simulink model "c00014M_harness"  (R2018a)
settings: Solver=ode3  StartTime=0.0  StopTime=10.0  RelTol=1e-3  EnableMultiTasking=on
undefined symbols (not defined in the file): b, DiscIntNeverNeededParam, J, K, L, PosMinimaW4, R, sigbuilder_block
(part 8 of 46)

== system c00014M_harness/M090 ==
  DW1 : Inport  OutMin=0  OutMax=4  OutDataTypeStr=int8
  DW2 : Inport  Port=2  OutMin=0  OutMax=4  OutDataTypeStr=int8
  DW4 : Inport  Port=3  OutMin=0  OutMax=4  OutDataTypeStr=int8
  P1W2 : Inport  Port=4  OutMin=0  OutMax=4  OutDataTypeStr=int8
  P3W4 : Inport  Port=5  OutMin=0  OutMax=4  OutDataTypeStr=int8
  P1W4 : Inport  Port=6  OutMin=0  OutMax=4  OutDataTypeStr=int8
  O1 : Inport  Port=7  OutDataTypeStr=boolean
  O2 : Inport  Port=8  OutDataTypeStr=boolean
  O4 : Inport  Port=9  OutDataTypeStr=boolean
  LD : Inport  Port=10  OutDataTypeStr=boolean
  CW1C : Inport  Port=11  OutMin=0  OutMax=4  OutDataTypeStr=int8
  CW2C : Inport  Port=12  OutMin=0  OutMax=4  OutDataTypeStr=int8
  CW4C : Inport  Port=13  OutMin=0  OutMax=4  OutDataTypeStr=int8
  Cyber : Subsystem
  M : Memory
  M1 : Memory
  M3 : Memory
  Physical : Subsystem
  S1 : Subsystem
  S2 : Subsystem
  S4 : Subsystem
  W1Pos : Outport
  W2Pos : Outport  Port=2
  W4Pos : Outport  Port=3
  wires:
  Cyber/3(W4) -> Physical/3(InW4)
  DW4/1 -> Cyber/6(DW4)
  Physical/3(W4) -> S4/1(PhyMeasure), W4Pos/1
  DW2/1 -> Cyber/5(DW2)
  P3W4/1 -> Cyber/8(P3W4)
  S2/1(SensorOut) -> M1/1
  Physical/2(W2) -> S2/1(PhyMeasure), W2Pos/1
  DW1/1 -> Cyber/4(DW1)
  M/1 -> Cyber/1(PosW1)
  M1/1 -> Cyber/2(PosW2)
  S4/1(SensorOut) -> M3/1
  CW1C/1 -> Cyber/14(CW1C)
  P1W4/1 -> Cyber/9(P1W4)
  P1W2/1 -> Cyber/7(P1W2)
  Cyber/2(W2) -> Physical/2(InW2)
  Cyber/1(W1) -> Physical/1(InW1)
  O1/1 -> Cyber/10(OW1)
  LD/1 -> Cyber/13(LD)
  O2/1 -> Cyber/11(OW2)
  O4/1 -> Cyber/12(OW4)
  Physical/1(W1) -> S1/1(PhyMeasure), W1Pos/1
  CW4C/1 -> Cyber/16(CW4C)
  CW2C/1 -> Cyber/15(CW2C)
  S1/1(SensorOut) -> M/1
  M3/1 -> Cyber/3(PosW4)

== system c00014M_harness/M091 ==
  DW1 : Inport  OutMin=0  OutMax=4  OutDataTypeStr=int8
  DW2 : Inport  Port=2  OutMin=0  OutMax=4  OutDataTypeStr=int8
  DW4 : Inport  Port=3  OutMin=0  OutMax=4  OutDataTypeStr=int8
  P1W2 : Inport  Port=4  OutMin=0  OutMax=4  OutDataTypeStr=int8
  P3W4 : Inport  Port=5  OutMin=0  OutMax=4  OutDataTypeStr=int8
  P1W4 : Inport  Port=6  OutMin=0  OutMax=4  OutDataTypeStr=int8
  O1 : Inport  Port=7  OutDataTypeStr=boolean
  O2 : Inport  Port=8  OutDataTypeStr=boolean
  O4 : Inport  Port=9  OutDataTypeStr=boolean
  LD : Inport  Port=10  OutDataTypeStr=boolean
  CW1C : Inport  Port=11  OutMin=0  OutMax=4  OutDataTypeStr=int8
  CW2C : Inport  Port=12  OutMin=0  OutMax=4  OutDataTypeStr=int8
  CW4C : Inport  Port=13  OutMin=0  OutMax=4  OutDataTypeStr=int8
  Cyber : Subsystem
  M : Memory
  M1 : Memory
  M3 : Memory
  Physical : Subsystem
  S1 : Subsystem
  S2 : Subsystem
  S4 : Subsystem
  W1Pos : Outport
  W2Pos : Outport  Port=2
  W4Pos : Outport  Port=3
  wires:
  Cyber/3(W4) -> Physical/3(InW4)
  DW4/1 -> Cyber/6(DW4)
  Physical/3(W4) -> S4/1(PhyMeasure), W4Pos/1
  DW2/1 -> Cyber/5(DW2)
  P3W4/1 -> Cyber/8(P3W4)
  S2/1(SensorOut) -> M1/1
  Physical/2(W2) -> S2/1(PhyMeasure), W2Pos/1
  DW1/1 -> Cyber/4(DW1)
  M/1 -> Cyber/1(PosW1)
  M1/1 -> Cyber/2(PosW2)
  S4/1(SensorOut) -> M3/1
  CW1C/1 -> Cyber/14(CW1C)
  P1W4/1 -> Cyber/9(P1W4)
  P1W2/1 -> Cyber/7(P1W2)
  Cyber/2(W2) -> Physical/2(InW2)
  Cyber/1(W1) -> Physical/1(InW1)
  O1/1 -> Cyber/10(OW1)
  LD/1 -> Cyber/13(LD)
  O2/1 -> Cyber/11(OW2)
  O4/1 -> Cyber/12(OW4)
  Physical/1(W1) -> S1/1(PhyMeasure), W1Pos/1
  CW4C/1 -> Cyber/16(CW4C)
  CW2C/1 -> Cyber/15(CW2C)
  S1/1(SensorOut) -> M/1
  M3/1 -> Cyber/3(PosW4)

== system c00014M_harness/M092 ==
  DW1 : Inport  OutMin=0  OutMax=4  OutDataTypeStr=int8
  DW2 : Inport  Port=2  OutMin=0  OutMax=4  OutDataTypeStr=int8
  DW4 : Inport  Port=3  OutMin=0  OutMax=4  OutDataTypeStr=int8
  P1W2 : Inport  Port=4  OutMin=0  OutMax=4  OutDataTypeStr=int8
  P3W4 : Inport  Port=5  OutMin=0  OutMax=4  OutDataTypeStr=int8
  P1W4 : Inport  Port=6  OutMin=0  OutMax=4  OutDataTypeStr=int8
  O1 : Inport  Port=7  OutDataTypeStr=boolean
  O2 : Inport  Port=8  OutDataTypeStr=boolean
  O4 : Inport  Port=9  OutDataTypeStr=boolean
  LD : Inport  Port=10  OutDataTypeStr=boolean
  CW1C : Inport  Port=11  OutMin=0  OutMax=4  OutDataTypeStr=int8
  CW2C : Inport  Port=12  OutMin=0  OutMax=4  OutDataTypeStr=int8
  CW4C : Inport  Port=13  OutMin=0  OutMax=4  OutDataTypeStr=int8
  Cyber : Subsystem
  M : Memory
  M1 : Memory
  M3 : Memory
  Physical : Subsystem
  S1 : Subsystem
  S2 : Subsystem
  S4 : Subsystem
  W1Pos : Outport
  W2Pos : Outport  Port=2
  W4Pos : Outport  Port=3
  wires:
  Cyber/3(W4) -> Physical/3(InW4)
  DW4/1 -> Cyber/6(DW4)
  Physical/3(W4) -> S4/1(PhyMeasure), W4Pos/1
  DW2/1 -> Cyber/5(DW2)
  P3W4/1 -> Cyber/8(P3W4)
  S2/1(SensorOut) -> M1/1
  Physical/2(W2) -> S2/1(PhyMeasure), W2Pos/1
  DW1/1 -> Cyber/4(DW1)
  M/1 -> Cyber/1(PosW1)
  M1/1 -> Cyber/2(PosW2)
  S4/1(SensorOut) -> M3/1
  CW1C/1 -> Cyber/14(CW1C)
  P1W4/1 -> Cyber/9(P1W4)
  P1W2/1 -> Cyber/7(P1W2)
  Cyber/2(W2) -> Physical/2(InW2)
  Cyber/1(W1) -> Physical/1(InW1)
  O1/1 -> Cyber/10(OW1)
  LD/1 -> Cyber/13(LD)
  O2/1 -> Cyber/11(OW2)
  O4/1 -> Cyber/12(OW4)
  Physical/1(W1) -> S1/1(PhyMeasure), W1Pos/1
  CW4C/1 -> Cyber/16(CW4C)
  CW2C/1 -> Cyber/15(CW2C)
  S1/1(SensorOut) -> M/1
  M3/1 -> Cyber/3(PosW4)

== system c00014M_harness/M094 ==
  DW1 : Inport  OutMin=0  OutMax=4  OutDataTypeStr=int8
  DW2 : Inport  Port=2  OutMin=0  OutMax=4  OutDataTypeStr=int8
  DW4 : Inport  Port=3  OutMin=0  OutMax=4  OutDataTypeStr=int8
  P1W2 : Inport  Port=4  OutMin=0  OutMax=4  OutDataTypeStr=int8
  P3W4 : Inport  Port=5  OutMin=0  OutMax=4  OutDataTypeStr=int8
  P1W4 : Inport  Port=6  OutMin=0  OutMax=4  OutDataTypeStr=int8
  O1 : Inport  Port=7  OutDataTypeStr=boolean
  O2 : Inport  Port=8  OutDataTypeStr=boolean
  O4 : Inport  Port=9  OutDataTypeStr=boolean
  LD : Inport  Port=10  OutDataTypeStr=boolean
  CW1C : Inport  Port=11  OutMin=0  OutMax=4  OutDataTypeStr=int8
  CW2C : Inport  Port=12  OutMin=0  OutMax=4  OutDataTypeStr=int8
  CW4C : Inport  Port=13  OutMin=0  OutMax=4  OutDataTypeStr=int8
  Cyber : Subsystem
  M : Memory
  M1 : Memory
  M3 : Memory
  Physical : Subsystem
  S1 : Subsystem
  S2 : Subsystem
  S4 : Subsystem
  W1Pos : Outport
  W2Pos : Outport  Port=2
  W4Pos : Outport  Port=3
  wires:
  Cyber/3(W4) -> Physical/3(InW4)
  DW4/1 -> Cyber/6(DW4)
  Physical/3(W4) -> S4/1(PhyMeasure), W4Pos/1
  DW2/1 -> Cyber/5(DW2)
  P3W4/1 -> Cyber/8(P3W4)
  S2/1(SensorOut) -> M1/1
  Physical/2(W2) -> S2/1(PhyMeasure), W2Pos/1
  DW1/1 -> Cyber/4(DW1)
  M/1 -> Cyber/1(PosW1)
  M1/1 -> Cyber/2(PosW2)
  S4/1(SensorOut) -> M3/1
  CW1C/1 -> Cyber/14(CW1C)
  P1W4/1 -> Cyber/9(P1W4)
  P1W2/1 -> Cyber/7(P1W2)
  Cyber/2(W2) -> Physical/2(InW2)
  Cyber/1(W1) -> Physical/1(InW1)
  O1/1 -> Cyber/10(OW1)
  LD/1 -> Cyber/13(LD)
  O2/1 -> Cyber/11(OW2)
  O4/1 -> Cyber/12(OW4)
  Physical/1(W1) -> S1/1(PhyMeasure), W1Pos/1
  CW4C/1 -> Cyber/16(CW4C)
  CW2C/1 -> Cyber/15(CW2C)
  S1/1(SensorOut) -> M/1
  M3/1 -> Cyber/3(PosW4)

== system c00014M_harness/M095 ==
  DW1 : Inport  OutMin=0  OutMax=4  OutDataTypeStr=int8
  DW2 : Inport  Port=2  OutMin=0  OutMax=4  OutDataTypeStr=int8
  DW4 : Inport  Port=3  OutMin=0  OutMax=4  OutDataTypeStr=int8
  P1W2 : Inport  Port=4  OutMin=0  OutMax=4  OutDataTypeStr=int8
  P3W4 : Inport  Port=5  OutMin=0  OutMax=4  OutDataTypeStr=int8
  P1W4 : Inport  Port=6  OutMin=0  OutMax=4  OutDataTypeStr=int8
  O1 : Inport  Port=7  OutDataTypeStr=boolean
  O2 : Inport  Port=8  OutDataTypeStr=boolean
  O4 : Inport  Port=9  OutDataTypeStr=boolean
  LD : Inport  Port=10  OutDataTypeStr=boolean
  CW1C : Inport  Port=11  OutMin=0  OutMax=4  OutDataTypeStr=int8
  CW2C : Inport  Port=12  OutMin=0  OutMax=4  OutDataTypeStr=int8
  CW4C : Inport  Port=13  OutMin=0  OutMax=4  OutDataTypeStr=int8
  Cyber : Subsystem
  M : Memory
  M1 : Memory
  M3 : Memory
  Physical : Subsystem
  S1 : Subsystem
  S2 : Subsystem
  S4 : Subsystem
  W1Pos : Outport
  W2Pos : Outport  Port=2
  W4Pos : Outport  Port=3
  wires:
  Cyber/3(W4) -> Physical/3(InW4)
  DW4/1 -> Cyber/6(DW4)
  Physical/3(W4) -> S4/1(PhyMeasure), W4Pos/1
  DW2/1 -> Cyber/5(DW2)
  P3W4/1 -> Cyber/8(P3W4)
  S2/1(SensorOut) -> M1/1
  Physical/2(W2) -> S2/1(PhyMeasure), W2Pos/1
  DW1/1 -> Cyber/4(DW1)
  M/1 -> Cyber/1(PosW1)
  M1/1 -> Cyber/2(PosW2)
  S4/1(SensorOut) -> M3/1
  CW1C/1 -> Cyber/14(CW1C)
  P1W4/1 -> Cyber/9(P1W4)
  P1W2/1 -> Cyber/7(P1W2)
  Cyber/2(W2) -> Physical/2(InW2)
  Cyber/1(W1) -> Physical/1(InW1)
  O1/1 -> Cyber/10(OW1)
  LD/1 -> Cyber/13(LD)
  O2/1 -> Cyber/11(OW2)
  O4/1 -> Cyber/12(OW4)
  Physical/1(W1) -> S1/1(PhyMeasure), W1Pos/1
  CW4C/1 -> Cyber/16(CW4C)
  CW2C/1 -> Cyber/15(CW2C)
  S1/1(SensorOut) -> M/1
  M3/1 -> Cyber/3(PosW4)

== system c00014M_harness/M096 ==
  DW1 : Inport  OutMin=0  OutMax=4  OutDataTypeStr=int8
  DW2 : Inport  Port=2  OutMin=0  OutMax=4  OutDataTypeStr=int8
  DW4 : Inport  Port=3  OutMin=0  OutMax=4  OutDataTypeStr=int8
  P1W2 : Inport  Port=4  OutMin=0  OutMax=4  OutDataTypeStr=int8
  P3W4 : Inport  Port=5  OutMin=0  OutMax=4  OutDataTypeStr=int8
  P1W4 : Inport  Port=6  OutMin=0  OutMax=4  OutDataTypeStr=int8
  O1 : Inport  Port=7  OutDataTypeStr=boolean
  O2 : Inport  Port=8  OutDataTypeStr=boolean
  O4 : Inport  Port=9  OutDataTypeStr=boolean
  LD : Inport  Port=10  OutDataTypeStr=boolean
  CW1C : Inport  Port=11  OutMin=0  OutMax=4  OutDataTypeStr=int8
  CW2C : Inport  Port=12  OutMin=0  OutMax=4  OutDataTypeStr=int8
  CW4C : Inport  Port=13  OutMin=0  OutMax=4  OutDataTypeStr=int8
  Cyber : Subsystem
  M : Memory
  M1 : Memory
  M3 : Memory
  Physical : Subsystem
  S1 : Subsystem
  S2 : Subsystem
  S4 : Subsystem
  W1Pos : Outport
  W2Pos : Outport  Port=2
  W4Pos : Outport  Port=3
  wires:
  Cyber/3(W4) -> Physical/3(InW4)
  DW4/1 -> Cyber/6(DW4)
  Physical/3(W4) -> S4/1(PhyMeasure), W4Pos/1
  DW2/1 -> Cyber/5(DW2)
  P3W4/1 -> Cyber/8(P3W4)
  S2/1(SensorOut) -> M1/1
  Physical/2(W2) -> S2/1(PhyMeasure), W2Pos/1
  DW1/1 -> Cyber/4(DW1)
  M/1 -> Cyber/1(PosW1)
  M1/1 -> Cyber/2(PosW2)
  S4/1(SensorOut) -> M3/1
  CW1C/1 -> Cyber/14(CW1C)
  P1W4/1 -> Cyber/9(P1W4)
  P1W2/1 -> Cyber/7(P1W2)
  Cyber/2(W2) -> Physical/2(InW2)
  Cyber/1(W1) -> Physical/1(InW1)
  O1/1 -> Cyber/10(OW1)
  LD/1 -> Cyber/13(LD)
  O2/1 -> Cyber/11(OW2)
  O4/1 -> Cyber/12(OW4)
  Physical/1(W1) -> S1/1(PhyMeasure), W1Pos/1
  CW4C/1 -> Cyber/16(CW4C)
  CW2C/1 -> Cyber/15(CW2C)
  S1/1(SensorOut) -> M/1
  M3/1 -> Cyber/3(PosW4)

== system c00014M_harness/M098 ==
  DW1 : Inport  OutMin=0  OutMax=4  OutDataTypeStr=int8
  DW2 : Inport  Port=2  OutMin=0  OutMax=4  OutDataTypeStr=int8
  DW4 : Inport  Port=3  OutMin=0  OutMax=4  OutDataTypeStr=int8
  P1W2 : Inport  Port=4  OutMin=0  OutMax=4  OutDataTypeStr=int8
  P3W4 : Inport  Port=5  OutMin=0  OutMax=4  OutDataTypeStr=int8
  P1W4 : Inport  Port=6  OutMin=0  OutMax=4  OutDataTypeStr=int8
  O1 : Inport  Port=7  OutDataTypeStr=boolean
  O2 : Inport  Port=8  OutDataTypeStr=boolean
  O4 : Inport  Port=9  OutDataTypeStr=boolean
  LD : Inport  Port=10  OutDataTypeStr=boolean
  CW1C : Inport  Port=11  OutMin=0  OutMax=4  OutDataTypeStr=int8
  CW2C : Inport  Port=12  OutMin=0  OutMax=4  OutDataTypeStr=int8
  CW4C : Inport  Port=13  OutMin=0  OutMax=4  OutDataTypeStr=int8
  Cyber : Subsystem
  M : Memory
  M1 : Memory
  M3 : Memory
  Physical : Subsystem
  S1 : Subsystem
  S2 : Subsystem
  S4 : Subsystem
  W1Pos : Outport
  W2Pos : Outport  Port=2
  W4Pos : Outport  Port=3
  wires:
  Cyber/3(W4) -> Physical/3(InW4)
  DW4/1 -> Cyber/6(DW4)
  Physical/3(W4) -> S4/1(PhyMeasure), W4Pos/1
  DW2/1 -> Cyber/5(DW2)
  P3W4/1 -> Cyber/8(P3W4)
  S2/1(SensorOut) -> M1/1
  Physical/2(W2) -> S2/1(PhyMeasure), W2Pos/1
  DW1/1 -> Cyber/4(DW1)
  M/1 -> Cyber/1(PosW1)
  M1/1 -> Cyber/2(PosW2)
  S4/1(SensorOut) -> M3/1
  CW1C/1 -> Cyber/14(CW1C)
  P1W4/1 -> Cyber/9(P1W4)
  P1W2/1 -> Cyber/7(P1W2)
  Cyber/2(W2) -> Physical/2(InW2)
  Cyber/1(W1) -> Physical/1(InW1)
  O1/1 -> Cyber/10(OW1)
  LD/1 -> Cyber/13(LD)
  O2/1 -> Cyber/11(OW2)
  O4/1 -> Cyber/12(OW4)
  Physical/1(W1) -> S1/1(PhyMeasure), W1Pos/1
  CW4C/1 -> Cyber/16(CW4C)
  CW2C/1 -> Cyber/15(CW2C)
  S1/1(SensorOut) -> M/1
  M3/1 -> Cyber/3(PosW4)

== system c00014M_harness/M099 ==
  DW1 : Inport  OutMin=0  OutMax=4  OutDataTypeStr=int8
  DW2 : Inport  Port=2  OutMin=0  OutMax=4  OutDataTypeStr=int8
  DW4 : Inport  Port=3  OutMin=0  OutMax=4  OutDataTypeStr=int8
  P1W2 : Inport  Port=4  OutMin=0  OutMax=4  OutDataTypeStr=int8
  P3W4 : Inport  Port=5  OutMin=0  OutMax=4  OutDataTypeStr=int8
  P1W4 : Inport  Port=6  OutMin=0  OutMax=4  OutDataTypeStr=int8
  O1 : Inport  Port=7  OutDataTypeStr=boolean
  O2 : Inport  Port=8  OutDataTypeStr=boolean
  O4 : Inport  Port=9  OutDataTypeStr=boolean
  LD : Inport  Port=10  OutDataTypeStr=boolean
  CW1C : Inport  Port=11  OutMin=0  OutMax=4  OutDataTypeStr=int8
  CW2C : Inport  Port=12  OutMin=0  OutMax=4  OutDataTypeStr=int8
  CW4C : Inport  Port=13  OutMin=0  OutMax=4  OutDataTypeStr=int8
  Cyber : Subsystem
  M : Memory
  M1 : Memory
  M3 : Memory
  Physical : Subsystem
  S1 : Subsystem
  S2 : Subsystem
  S4 : Subsystem
  W1Pos : Outport
  W2Pos : Outport  Port=2
  W4Pos : Outport  Port=3
  wires:
  Cyber/3(W4) -> Physical/3(InW4)
  DW4/1 -> Cyber/6(DW4)
  Physical/3(W4) -> S4/1(PhyMeasure), W4Pos/1
  DW2/1 -> Cyber/5(DW2)
  P3W4/1 -> Cyber/8(P3W4)
  S2/1(SensorOut) -> M1/1
  Physical/2(W2) -> S2/1(PhyMeasure), W2Pos/1
  DW1/1 -> Cyber/4(DW1)
  M/1 -> Cyber/1(PosW1)
  M1/1 -> Cyber/2(PosW2)
  S4/1(SensorOut) -> M3/1
  CW1C/1 -> Cyber/14(CW1C)
  P1W4/1 -> Cyber/9(P1W4)
  P1W2/1 -> Cyber/7(P1W2)
  Cyber/2(W2) -> Physical/2(InW2)
  Cyber/1(W1) -> Physical/1(InW1)
  O1/1 -> Cyber/10(OW1)
  LD/1 -> Cyber/13(LD)
  O2/1 -> Cyber/11(OW2)
  O4/1 -> Cyber/12(OW4)
  Physical/1(W1) -> S1/1(PhyMeasure), W1Pos/1
  CW4C/1 -> Cyber/16(CW4C)
  CW2C/1 -> Cyber/15(CW2C)
  S1/1(SensorOut) -> M/1
  M3/1 -> Cyber/3(PosW4)

== system c00014M_harness/M100 ==
  DW1 : Inport  OutMin=0  OutMax=4  OutDataTypeStr=int8
  DW2 : Inport  Port=2  OutMin=0  OutMax=4  OutDataTypeStr=int8
  DW4 : Inport  Port=3  OutMin=0  OutMax=4  OutDataTypeStr=int8
  P1W2 : Inport  Port=4  OutMin=0  OutMax=4  OutDataTypeStr=int8
  P3W4 : Inport  Port=5  OutMin=0  OutMax=4  OutDataTypeStr=int8
  P1W4 : Inport  Port=6  OutMin=0  OutMax=4  OutDataTypeStr=int8
  O1 : Inport  Port=7  OutDataTypeStr=boolean
  O2 : Inport  Port=8  OutDataTypeStr=boolean
  O4 : Inport  Port=9  OutDataTypeStr=boolean
  LD : Inport  Port=10  OutDataTypeStr=boolean
  CW1C : Inport  Port=11  OutMin=0  OutMax=4  OutDataTypeStr=int8
  CW2C : Inport  Port=12  OutMin=0  OutMax=4  OutDataTypeStr=int8
  CW4C : Inport  Port=13  OutMin=0  OutMax=4  OutDataTypeStr=int8
  Cyber : Subsystem
  M : Memory
  M1 : Memory
  M3 : Memory
  Physical : Subsystem
  S1 : Subsystem
  S2 : Subsystem
  S4 : Subsystem
  W1Pos : Outport
  W2Pos : Outport  Port=2
  W4Pos : Outport  Port=3
  wires:
  Cyber/3(W4) -> Physical/3(InW4)
  DW4/1 -> Cyber/6(DW4)
  Physical/3(W4) -> S4/1(PhyMeasure), W4Pos/1
  DW2/1 -> Cyber/5(DW2)
  P3W4/1 -> Cyber/8(P3W4)
  S2/1(SensorOut) -> M1/1
  Physical/2(W2) -> S2/1(PhyMeasure), W2Pos/1
  DW1/1 -> Cyber/4(DW1)
  M/1 -> Cyber/1(PosW1)
  M1/1 -> Cyber/2(PosW2)
  S4/1(SensorOut) -> M3/1
  CW1C/1 -> Cyber/14(CW1C)
  P1W4/1 -> Cyber/9(P1W4)
  P1W2/1 -> Cyber/7(P1W2)
  Cyber/2(W2) -> Physical/2(InW2)
  Cyber/1(W1) -> Physical/1(InW1)
  O1/1 -> Cyber/10(OW1)
  LD/1 -> Cyber/13(LD)
  O2/1 -> Cyber/11(OW2)
  O4/1 -> Cyber/12(OW4)
  Physical/1(W1) -> S1/1(PhyMeasure), W1Pos/1
  CW4C/1 -> Cyber/16(CW4C)
  CW2C/1 -> Cyber/15(CW2C)
  S1/1(SensorOut) -> M/1
  M3/1 -> Cyber/3(PosW4)

== system c00014M_harness/M102 ==
  DW1 : Inport  OutMin=0  OutMax=4  OutDataTypeStr=int8
  DW2 : Inport  Port=2  OutMin=0  OutMax=4  OutDataTypeStr=int8
  DW4 : Inport  Port=3  OutMin=0  OutMax=4  OutDataTypeStr=int8
  P1W2 : Inport  Port=4  OutMin=0  OutMax=4  OutDataTypeStr=int8
  P3W4 : Inport  Port=5  OutMin=0  OutMax=4  OutDataTypeStr=int8
  P1W4 : Inport  Port=6  OutMin=0  OutMax=4  OutDataTypeStr=int8
  O1 : Inport  Port=7  OutDataTypeStr=boolean
  O2 : Inport  Port=8  OutDataTypeStr=boolean
  O4 : Inport  Port=9  OutDataTypeStr=boolean
  LD : Inport  Port=10  OutDataTypeStr=boolean
  CW1C : Inport  Port=11  OutMin=0  OutMax=4  OutDataTypeStr=int8
  CW2C : Inport  Port=12  OutMin=0  OutMax=4  OutDataTypeStr=int8
  CW4C : Inport  Port=13  OutMin=0  OutMax=4  OutDataTypeStr=int8
  Cyber : Subsystem
  M : Memory
  M1 : Memory
  M3 : Memory
  Physical : Subsystem
  S1 : Subsystem
  S2 : Subsystem
  S4 : Subsystem
  W1Pos : Outport
  W2Pos : Outport  Port=2
  W4Pos : Outport  Port=3
  wires:
  Cyber/3(W4) -> Physical/3(InW4)
  DW4/1 -> Cyber/6(DW4)
  Physical/3(W4) -> S4/1(PhyMeasure), W4Pos/1
  DW2/1 -> Cyber/5(DW2)
  P3W4/1 -> Cyber/8(P3W4)
  S2/1(SensorOut) -> M1/1
  Physical/2(W2) -> S2/1(PhyMeasure), W2Pos/1
  DW1/1 -> Cyber/4(DW1)
  M/1 -> Cyber/1(PosW1)
  M1/1 -> Cyber/2(PosW2)
  S4/1(SensorOut) -> M3/1
  CW1C/1 -> Cyber/14(CW1C)
  P1W4/1 -> Cyber/9(P1W4)
  P1W2/1 -> Cyber/7(P1W2)
  Cyber/2(W2) -> Physical/2(InW2)
  Cyber/1(W1) -> Physical/1(InW1)
  O1/1 -> Cyber/10(OW1)
  LD/1 -> Cyber/13(LD)
  O2/1 -> Cyber/11(OW2)
  O4/1 -> Cyber/12(OW4)
  Physical/1(W1) -> S1/1(PhyMeasure), W1Pos/1
  CW4C/1 -> Cyber/16(CW4C)
  CW2C/1 -> Cyber/15(CW2C)
  S1/1(SensorOut) -> M/1
  M3/1 -> Cyber/3(PosW4)

== system c00014M_harness/M103 ==
  DW1 : Inport  OutMin=0  OutMax=4  OutDataTypeStr=int8
  DW2 : Inport  Port=2  OutMin=0  OutMax=4  OutDataTypeStr=int8
  DW4 : Inport  Port=3  OutMin=0  OutMax=4  OutDataTypeStr=int8
  P1W2 : Inport  Port=4  OutMin=0  OutMax=4  OutDataTypeStr=int8
  P3W4 : Inport  Port=5  OutMin=0  OutMax=4  OutDataTypeStr=int8
  P1W4 : Inport  Port=6  OutMin=0  OutMax=4  OutDataTypeStr=int8
  O1 : Inport  Port=7  OutDataTypeStr=boolean
  O2 : Inport  Port=8  OutDataTypeStr=boolean
  O4 : Inport  Port=9  OutDataTypeStr=boolean
  LD : Inport  Port=10  OutDataTypeStr=boolean
  CW1C : Inport  Port=11  OutMin=0  OutMax=4  OutDataTypeStr=int8
  CW2C : Inport  Port=12  OutMin=0  OutMax=4  OutDataTypeStr=int8
  CW4C : Inport  Port=13  OutMin=0  OutMax=4  OutDataTypeStr=int8
  Cyber : Subsystem
  M : Memory
  M1 : Memory
  M3 : Memory
  Physical : Subsystem
  S1 : Subsystem
  S2 : Subsystem
  S4 : Subsystem
  W1Pos : Outport
  W2Pos : Outport  Port=2
  W4Pos : Outport  Port=3
  wires:
  Cyber/3(W4) -> Physical/3(InW4)
  DW4/1 -> Cyber/6(DW4)
  Physical/3(W4) -> S4/1(PhyMeasure), W4Pos/1
  DW2/1 -> Cyber/5(DW2)
  P3W4/1 -> Cyber/8(P3W4)
  S2/1(SensorOut) -> M1/1
  Physical/2(W2) -> S2/1(PhyMeasure), W2Pos/1
  DW1/1 -> Cyber/4(DW1)
  M/1 -> Cyber/1(PosW1)
  M1/1 -> Cyber/2(PosW2)
  S4/1(SensorOut) -> M3/1
  CW1C/1 -> Cyber/14(CW1C)
  P1W4/1 -> Cyber/9(P1W4)
  P1W2/1 -> Cyber/7(P1W2)
  Cyber/2(W2) -> Physical/2(InW2)
  Cyber/1(W1) -> Physical/1(InW1)
  O1/1 -> Cyber/10(OW1)
  LD/1 -> Cyber/13(LD)
  O2/1 -> Cyber/11(OW2)
  O4/1 -> Cyber/12(OW4)
  Physical/1(W1) -> S1/1(PhyMeasure), W1Pos/1
  CW4C/1 -> Cyber/16(CW4C)
  CW2C/1 -> Cyber/15(CW2C)
  S1/1(SensorOut) -> M/1
  M3/1 -> Cyber/3(PosW4)

== system c00014M_harness/M104 ==
  DW1 : Inport  OutMin=0  OutMax=4  OutDataTypeStr=int8
  DW2 : Inport  Port=2  OutMin=0  OutMax=4  OutDataTypeStr=int8
  DW4 : Inport  Port=3  OutMin=0  OutMax=4  OutDataTypeStr=int8
  P1W2 : Inport  Port=4  OutMin=0  OutMax=4  OutDataTypeStr=int8
  P3W4 : Inport  Port=5  OutMin=0  OutMax=4  OutDataTypeStr=int8
  P1W4 : Inport  Port=6  OutMin=0  OutMax=4  OutDataTypeStr=int8
  O1 : Inport  Port=7  OutDataTypeStr=boolean
  O2 : Inport  Port=8  OutDataTypeStr=boolean
  O4 : Inport  Port=9  OutDataTypeStr=boolean
  LD : Inport  Port=10  OutDataTypeStr=boolean
  CW1C : Inport  Port=11  OutMin=0  OutMax=4  OutDataTypeStr=int8
  CW2C : Inport  Port=12  OutMin=0  OutMax=4  OutDataTypeStr=int8
  CW4C : Inport  Port=13  OutMin=0  OutMax=4  OutDataTypeStr=int8
  Cyber : Subsystem
  M : Memory
  M1 : Memory
  M3 : Memory
  Physical : Subsystem
  S1 : Subsystem
  S2 : Subsystem
  S4 : Subsystem
  W1Pos : Outport
  W2Pos : Outport  Port=2
  W4Pos : Outport  Port=3
  wires:
  Cyber/3(W4) -> Physical/3(InW4)
  DW4/1 -> Cyber/6(DW4)
  Physical/3(W4) -> S4/1(PhyMeasure), W4Pos/1
  DW2/1 -> Cyber/5(DW2)
  P3W4/1 -> Cyber/8(P3W4)
  S2/1(SensorOut) -> M1/1
  Physical/2(W2) -> S2/1(PhyMeasure), W2Pos/1
  DW1/1 -> Cyber/4(DW1)
  M/1 -> Cyber/1(PosW1)
  M1/1 -> Cyber/2(PosW2)
  S4/1(SensorOut) -> M3/1
  CW1C/1 -> Cyber/14(CW1C)
  P1W4/1 -> Cyber/9(P1W4)
  P1W2/1 -> Cyber/7(P1W2)
  Cyber/2(W2) -> Physical/2(InW2)
  Cyber/1(W1) -> Physical/1(InW1)
  O1/1 -> Cyber/10(OW1)
  LD/1 -> Cyber/13(LD)
  O2/1 -> Cyber/11(OW2)
  O4/1 -> Cyber/12(OW4)
  Physical/1(W1) -> S1/1(PhyMeasure), W1Pos/1
  CW4C/1 -> Cyber/16(CW4C)
  CW2C/1 -> Cyber/15(CW2C)
  S1/1(SensorOut) -> M/1
  M3/1 -> Cyber/3(PosW4)

== system c00014M_harness/M106 ==
  DW1 : Inport  OutMin=0  OutMax=4  OutDataTypeStr=int8
  DW2 : Inport  Port=2  OutMin=0  OutMax=4  OutDataTypeStr=int8
  DW4 : Inport  Port=3  OutMin=0  OutMax=4  OutDataTypeStr=int8
  P1W2 : Inport  Port=4  OutMin=0  OutMax=4  OutDataTypeStr=int8
  P3W4 : Inport  Port=5  OutMin=0  OutMax=4  OutDataTypeStr=int8
  P1W4 : Inport  Port=6  OutMin=0  OutMax=4  OutDataTypeStr=int8
  O1 : Inport  Port=7  OutDataTypeStr=boolean
  O2 : Inport  Port=8  OutDataTypeStr=boolean
  O4 : Inport  Port=9  OutDataTypeStr=boolean
  LD : Inport  Port=10  OutDataTypeStr=boolean
  CW1C : Inport  Port=11  OutMin=0  OutMax=4  OutDataTypeStr=int8
  CW2C : Inport  Port=12  OutMin=0  OutMax=4  OutDataTypeStr=int8
  CW4C : Inport  Port=13  OutMin=0  OutMax=4  OutDataTypeStr=int8
  Cyber : Subsystem
  M : Memory
  M1 : Memory
  M3 : Memory
  Physical : Subsystem
  S1 : Subsystem
  S2 : Subsystem
  S4 : Subsystem
  W1Pos : Outport
  W2Pos : Outport  Port=2
  W4Pos : Outport  Port=3
  wires:
  Cyber/3(W4) -> Physical/3(InW4)
  DW4/1 -> Cyber/6(DW4)
  Physical/3(W4) -> S4/1(PhyMeasure), W4Pos/1
  DW2/1 -> Cyber/5(DW2)
  P3W4/1 -> Cyber/8(P3W4)
  S2/1(SensorOut) -> M1/1
  Physical/2(W2) -> S2/1(PhyMeasure), W2Pos/1
  DW1/1 -> Cyber/4(DW1)
  M/1 -> Cyber/1(PosW1)
  M1/1 -> Cyber/2(PosW2)
  S4/1(SensorOut) -> M3/1
  CW1C/1 -> Cyber/14(CW1C)
  P1W4/1 -> Cyber/9(P1W4)
  P1W2/1 -> Cyber/7(P1W2)
  Cyber/2(W2) -> Physical/2(InW2)
  Cyber/1(W1) -> Physical/1(InW1)
  O1/1 -> Cyber/10(OW1)
  LD/1 -> Cyber/13(LD)
  O2/1 -> Cyber/11(OW2)
  O4/1 -> Cyber/12(OW4)
  Physical/1(W1) -> S1/1(PhyMeasure), W1Pos/1
  CW4C/1 -> Cyber/16(CW4C)
  CW2C/1 -> Cyber/15(CW2C)
  S1/1(SensorOut) -> M/1
  M3/1 -> Cyber/3(PosW4)

== system c00014M_harness/M107 ==
  DW1 : Inport  OutMin=0  OutMax=4  OutDataTypeStr=int8
  DW2 : Inport  Port=2  OutMin=0  OutMax=4  OutDataTypeStr=int8
  DW4 : Inport  Port=3  OutMin=0  OutMax=4  OutDataTypeStr=int8
  P1W2 : Inport  Port=4  OutMin=0  OutMax=4  OutDataTypeStr=int8
  P3W4 : Inport  Port=5  OutMin=0  OutMax=4  OutDataTypeStr=int8
  P1W4 : Inport  Port=6  OutMin=0  OutMax=4  OutDataTypeStr=int8
  O1 : Inport  Port=7  OutDataTypeStr=boolean
  O2 : Inport  Port=8  OutDataTypeStr=boolean
  O4 : Inport  Port=9  OutDataTypeStr=boolean
  LD : Inport  Port=10  OutDataTypeStr=boolean
  CW1C : Inport  Port=11  OutMin=0  OutMax=4  OutDataTypeStr=int8
  CW2C : Inport  Port=12  OutMin=0  OutMax=4  OutDataTypeStr=int8
  CW4C : Inport  Port=13  OutMin=0  OutMax=4  OutDataTypeStr=int8
  Cyber : Subsystem
  M : Memory
  M1 : Memory
  M3 : Memory
  Physical : Subsystem
  S1 : Subsystem
  S2 : Subsystem
  S4 : Subsystem
  W1Pos : Outport
  W2Pos : Outport  Port=2
  W4Pos : Outport  Port=3
  wires:
  Cyber/3(W4) -> Physical/3(InW4)
  DW4/1 -> Cyber/6(DW4)
  Physical/3(W4) -> S4/1(PhyMeasure), W4Pos/1
  DW2/1 -> Cyber/5(DW2)
  P3W4/1 -> Cyber/8(P3W4)
  S2/1(SensorOut) -> M1/1
  Physical/2(W2) -> S2/1(PhyMeasure), W2Pos/1
  DW1/1 -> Cyber/4(DW1)
  M/1 -> Cyber/1(PosW1)
  M1/1 -> Cyber/2(PosW2)
  S4/1(SensorOut) -> M3/1
  CW1C/1 -> Cyber/14(CW1C)
  P1W4/1 -> Cyber/9(P1W4)
  P1W2/1 -> Cyber/7(P1W2)
  Cyber/2(W2) -> Physical/2(InW2)
  Cyber/1(W1) -> Physical/1(InW1)
  O1/1 -> Cyber/10(OW1)
  LD/1 -> Cyber/13(LD)
  O2/1 -> Cyber/11(OW2)
  O4/1 -> Cyber/12(OW4)
  Physical/1(W1) -> S1/1(PhyMeasure), W1Pos/1
  CW4C/1 -> Cyber/16(CW4C)
  CW2C/1 -> Cyber/15(CW2C)
  S1/1(SensorOut) -> M/1
  M3/1 -> Cyber/3(PosW4)

== system c00014M_harness/M108 ==
  DW1 : Inport  OutMin=0  OutMax=4  OutDataTypeStr=int8
  DW2 : Inport  Port=2  OutMin=0  OutMax=4  OutDataTypeStr=int8
  DW4 : Inport  Port=3  OutMin=0  OutMax=4  OutDataTypeStr=int8
  P1W2 : Inport  Port=4  OutMin=0  OutMax=4  OutDataTypeStr=int8
  P3W4 : Inport  Port=5  OutMin=0  OutMax=4  OutDataTypeStr=int8
  P1W4 : Inport  Port=6  OutMin=0  OutMax=4  OutDataTypeStr=int8
  O1 : Inport  Port=7  OutDataTypeStr=boolean
  O2 : Inport  Port=8  OutDataTypeStr=boolean
  O4 : Inport  Port=9  OutDataTypeStr=boolean
  LD : Inport  Port=10  OutDataTypeStr=boolean
  CW1C : Inport  Port=11  OutMin=0  OutMax=4  OutDataTypeStr=int8
  CW2C : Inport  Port=12  OutMin=0  OutMax=4  OutDataTypeStr=int8
  CW4C : Inport  Port=13  OutMin=0  OutMax=4  OutDataTypeStr=int8
  Cyber : Subsystem
  M : Memory
  M1 : Memory
  M3 : Memory
  Physical : Subsystem
  S1 : Subsystem
  S2 : Subsystem
  S4 : Subsystem
  W1Pos : Outport
  W2Pos : Outport  Port=2
  W4Pos : Outport  Port=3
  wires:
  Cyber/3(W4) -> Physical/3(InW4)
  DW4/1 -> Cyber/6(DW4)
  Physical/3(W4) -> S4/1(PhyMeasure), W4Pos/1
  DW2/1 -> Cyber/5(DW2)
  P3W4/1 -> Cyber/8(P3W4)
  S2/1(SensorOut) -> M1/1
  Physical/2(W2) -> S2/1(PhyMeasure), W2Pos/1
  DW1/1 -> Cyber/4(DW1)
  M/1 -> Cyber/1(PosW1)
  M1/1 -> Cyber/2(PosW2)
  S4/1(SensorOut) -> M3/1
  CW1C/1 -> Cyber/14(CW1C)
  P1W4/1 -> Cyber/9(P1W4)
  P1W2/1 -> Cyber/7(P1W2)
  Cyber/2(W2) -> Physical/2(InW2)
  Cyber/1(W1) -> Physical/1(InW1)
  O1/1 -> Cyber/10(OW1)
  LD/1 -> Cyber/13(LD)
  O2/1 -> Cyber/11(OW2)
  O4/1 -> Cyber/12(OW4)
  Physical/1(W1) -> S1/1(PhyMeasure), W1Pos/1
  CW4C/1 -> Cyber/16(CW4C)
  CW2C/1 -> Cyber/15(CW2C)
  S1/1(SensorOut) -> M/1
  M3/1 -> Cyber/3(PosW4)

== system c00014M_harness/M110 ==
  DW1 : Inport  OutMin=0  OutMax=4  OutDataTypeStr=int8
  DW2 : Inport  Port=2  OutMin=0  OutMax=4  OutDataTypeStr=int8
  DW4 : Inport  Port=3  OutMin=0  OutMax=4  OutDataTypeStr=int8
  P1W2 : Inport  Port=4  OutMin=0  OutMax=4  OutDataTypeStr=int8
  P3W4 : Inport  Port=5  OutMin=0  OutMax=4  OutDataTypeStr=int8
  P1W4 : Inport  Port=6  OutMin=0  OutMax=4  OutDataTypeStr=int8
  O1 : Inport  Port=7  OutDataTypeStr=boolean
  O2 : Inport  Port=8  OutDataTypeStr=boolean
  O4 : Inport  Port=9  OutDataTypeStr=boolean
  LD : Inport  Port=10  OutDataTypeStr=boolean
  CW1C : Inport  Port=11  OutMin=0  OutMax=4  OutDataTypeStr=int8
  CW2C : Inport  Port=12  OutMin=0  OutMax=4  OutDataTypeStr=int8
  CW4C : Inport  Port=13  OutMin=0  OutMax=4  OutDataTypeStr=int8
  Cyber : Subsystem
  M : Memory
  M1 : Memory
  M3 : Memory
  Physical : Subsystem
  S1 : Subsystem
  S2 : Subsystem
  S4 : Subsystem
  W1Pos : Outport
  W2Pos : Outport  Port=2
  W4Pos : Outport  Port=3
  wires:
  Cyber/3(W4) -> Physical/3(InW4)
  DW4/1 -> Cyber/6(DW4)
  Physical/3(W4) -> S4/1(PhyMeasure), W4Pos/1
  DW2/1 -> Cyber/5(DW2)
  P3W4/1 -> Cyber/8(P3W4)
  S2/1(SensorOut) -> M1/1
  Physical/2(W2) -> S2/1(PhyMeasure), W2Pos/1
  DW1/1 -> Cyber/4(DW1)
  M/1 -> Cyber/1(PosW1)
  M1/1 -> Cyber/2(PosW2)
  S4/1(SensorOut) -> M3/1
  CW1C/1 -> Cyber/14(CW1C)
  P1W4/1 -> Cyber/9(P1W4)
  P1W2/1 -> Cyber/7(P1W2)
  Cyber/2(W2) -> Physical/2(InW2)
  Cyber/1(W1) -> Physical/1(InW1)
  O1/1 -> Cyber/10(OW1)
  LD/1 -> Cyber/13(LD)
  O2/1 -> Cyber/11(OW2)
  O4/1 -> Cyber/12(OW4)
  Physical/1(W1) -> S1/1(PhyMeasure), W1Pos/1
  CW4C/1 -> Cyber/16(CW4C)
  CW2C/1 -> Cyber/15(CW2C)
  S1/1(SensorOut) -> M/1
  M3/1 -> Cyber/3(PosW4)

== system c00014M_harness/M111 ==
  DW1 : Inport  OutMin=0  OutMax=4  OutDataTypeStr=int8
  DW2 : Inport  Port=2  OutMin=0  OutMax=4  OutDataTypeStr=int8
  DW4 : Inport  Port=3  OutMin=0  OutMax=4  OutDataTypeStr=int8
  P1W2 : Inport  Port=4  OutMin=0  OutMax=4  OutDataTypeStr=int8
  P3W4 : Inport  Port=5  OutMin=0  OutMax=4  OutDataTypeStr=int8
  P1W4 : Inport  Port=6  OutMin=0  OutMax=4  OutDataTypeStr=int8
  O1 : Inport  Port=7  OutDataTypeStr=boolean
  O2 : Inport  Port=8  OutDataTypeStr=boolean
  O4 : Inport  Port=9  OutDataTypeStr=boolean
  LD : Inport  Port=10  OutDataTypeStr=boolean
  CW1C : Inport  Port=11  OutMin=0  OutMax=4  OutDataTypeStr=int8
  CW2C : Inport  Port=12  OutMin=0  OutMax=4  OutDataTypeStr=int8
  CW4C : Inport  Port=13  OutMin=0  OutMax=4  OutDataTypeStr=int8
  Cyber : Subsystem
  M : Memory
  M1 : Memory
  M3 : Memory
  Physical : Subsystem
  S1 : Subsystem
  S2 : Subsystem
  S4 : Subsystem
  W1Pos : Outport
  W2Pos : Outport  Port=2
  W4Pos : Outport  Port=3
  wires:
  Cyber/3(W4) -> Physical/3(InW4)
  DW4/1 -> Cyber/6(DW4)
  Physical/3(W4) -> S4/1(PhyMeasure), W4Pos/1
  DW2/1 -> Cyber/5(DW2)
  P3W4/1 -> Cyber/8(P3W4)
  S2/1(SensorOut) -> M1/1
  Physical/2(W2) -> S2/1(PhyMeasure), W2Pos/1
  DW1/1 -> Cyber/4(DW1)
  M/1 -> Cyber/1(PosW1)
  M1/1 -> Cyber/2(PosW2)
  S4/1(SensorOut) -> M3/1
  CW1C/1 -> Cyber/14(CW1C)
  P1W4/1 -> Cyber/9(P1W4)
  P1W2/1 -> Cyber/7(P1W2)
  Cyber/2(W2) -> Physical/2(InW2)
  Cyber/1(W1) -> Physical/1(InW1)
  O1/1 -> Cyber/10(OW1)
  LD/1 -> Cyber/13(LD)
  O2/1 -> Cyber/11(OW2)
  O4/1 -> Cyber/12(OW4)
  Physical/1(W1) -> S1/1(PhyMeasure), W1Pos/1
  CW4C/1 -> Cyber/16(CW4C)
  CW2C/1 -> Cyber/15(CW2C)
  S1/1(SensorOut) -> M/1
  M3/1 -> Cyber/3(PosW4)

== system c00014M_harness/M112 ==
  DW1 : Inport  OutMin=0  OutMax=4  OutDataTypeStr=int8
  DW2 : Inport  Port=2  OutMin=0  OutMax=4  OutDataTypeStr=int8
  DW4 : Inport  Port=3  OutMin=0  OutMax=4  OutDataTypeStr=int8
  P1W2 : Inport  Port=4  OutMin=0  OutMax=4  OutDataTypeStr=int8
  P3W4 : Inport  Port=5  OutMin=0  OutMax=4  OutDataTypeStr=int8
  P1W4 : Inport  Port=6  OutMin=0  OutMax=4  OutDataTypeStr=int8
  O1 : Inport  Port=7  OutDataTypeStr=boolean
  O2 : Inport  Port=8  OutDataTypeStr=boolean
  O4 : Inport  Port=9  OutDataTypeStr=boolean
  LD : Inport  Port=10  OutDataTypeStr=boolean
  CW1C : Inport  Port=11  OutMin=0  OutMax=4  OutDataTypeStr=int8
  CW2C : Inport  Port=12  OutMin=0  OutMax=4  OutDataTypeStr=int8
  CW4C : Inport  Port=13  OutMin=0  OutMax=4  OutDataTypeStr=int8
  Cyber : Subsystem
  M : Memory
  M1 : Memory
  M3 : Memory
  Physical : Subsystem
  S1 : Subsystem
  S2 : Subsystem
  S4 : Subsystem
  W1Pos : Outport
  W2Pos : Outport  Port=2
  W4Pos : Outport  Port=3
  wires:
  Cyber/3(W4) -> Physical/3(InW4)
  DW4/1 -> Cyber/6(DW4)
  Physical/3(W4) -> S4/1(PhyMeasure), W4Pos/1
  DW2/1 -> Cyber/5(DW2)
  P3W4/1 -> Cyber/8(P3W4)
  S2/1(SensorOut) -> M1/1
  Physical/2(W2) -> S2/1(PhyMeasure), W2Pos/1
  DW1/1 -> Cyber/4(DW1)
  M/1 -> Cyber/1(PosW1)
  M1/1 -> Cyber/2(PosW2)
  S4/1(SensorOut) -> M3/1
  CW1C/1 -> Cyber/14(CW1C)
  P1W4/1 -> Cyber/9(P1W4)
  P1W2/1 -> Cyber/7(P1W2)
  Cyber/2(W2) -> Physical/2(InW2)
  Cyber/1(W1) -> Physical/1(InW1)
  O1/1 -> Cyber/10(OW1)
  LD/1 -> Cyber/13(LD)
  O2/1 -> Cyber/11(OW2)
  O4/1 -> Cyber/12(OW4)
  Physical/1(W1) -> S1/1(PhyMeasure), W1Pos/1
  CW4C/1 -> Cyber/16(CW4C)
  CW2C/1 -> Cyber/15(CW2C)
  S1/1(SensorOut) -> M/1
  M3/1 -> Cyber/3(PosW4)

== system c00014M_harness/M114 ==
  DW1 : Inport  OutMin=0  OutMax=4  OutDataTypeStr=int8
  DW2 : Inport  Port=2  OutMin=0  OutMax=4  OutDataTypeStr=int8
  DW4 : Inport  Port=3  OutMin=0  OutMax=4  OutDataTypeStr=int8
  P1W2 : Inport  Port=4  OutMin=0  OutMax=4  OutDataTypeStr=int8
  P3W4 : Inport  Port=5  OutMin=0  OutMax=4  OutDataTypeStr=int8
  P1W4 : Inport  Port=6  OutMin=0  OutMax=4  OutDataTypeStr=int8
  O1 : Inport  Port=7  OutDataTypeStr=boolean
  O2 : Inport  Port=8  OutDataTypeStr=boolean
  O4 : Inport  Port=9  OutDataTypeStr=boolean
  LD : Inport  Port=10  OutDataTypeStr=boolean
  CW1C : Inport  Port=11  OutMin=0  OutMax=4  OutDataTypeStr=int8
  CW2C : Inport  Port=12  OutMin=0  OutMax=4  OutDataTypeStr=int8
  CW4C : Inport  Port=13  OutMin=0  OutMax=4  OutDataTypeStr=int8
  Cyber : Subsystem
  M : Memory
  M1 : Memory
  M3 : Memory
  Physical : Subsystem
  S1 : Subsystem
  S2 : Subsystem
  S4 : Subsystem
  W1Pos : Outport
  W2Pos : Outport  Port=2
  W4Pos : Outport  Port=3
  wires:
  Cyber/3(W4) -> Physical/3(InW4)
  DW4/1 -> Cyber/6(DW4)
  Physical/3(W4) -> S4/1(PhyMeasure), W4Pos/1
  DW2/1 -> Cyber/5(DW2)
  P3W4/1 -> Cyber/8(P3W4)
  S2/1(SensorOut) -> M1/1
  Physical/2(W2) -> S2/1(PhyMeasure), W2Pos/1
  DW1/1 -> Cyber/4(DW1)
  M/1 -> Cyber/1(PosW1)
  M1/1 -> Cyber/2(PosW2)
  S4/1(SensorOut) -> M3/1
  CW1C/1 -> Cyber/14(CW1C)
  P1W4/1 -> Cyber/9(P1W4)
  P1W2/1 -> Cyber/7(P1W2)
  Cyber/2(W2) -> Physical/2(InW2)
  Cyber/1(W1) -> Physical/1(InW1)
  O1/1 -> Cyber/10(OW1)
  LD/1 -> Cyber/13(LD)
  O2/1 -> Cyber/11(OW2)
  O4/1 -> Cyber/12(OW4)
  Physical/1(W1) -> S1/1(PhyMeasure), W1Pos/1
  CW4C/1 -> Cyber/16(CW4C)
  CW2C/1 -> Cyber/15(CW2C)
  S1/1(SensorOut) -> M/1
  M3/1 -> Cyber/3(PosW4)

== system c00014M_harness/M115 ==
  DW1 : Inport  OutMin=0  OutMax=4  OutDataTypeStr=int8
  DW2 : Inport  Port=2  OutMin=0  OutMax=4  OutDataTypeStr=int8
  DW4 : Inport  Port=3  OutMin=0  OutMax=4  OutDataTypeStr=int8
  P1W2 : Inport  Port=4  OutMin=0  OutMax=4  OutDataTypeStr=int8
  P3W4 : Inport  Port=5  OutMin=0  OutMax=4  OutDataTypeStr=int8
  P1W4 : Inport  Port=6  OutMin=0  OutMax=4  OutDataTypeStr=int8
  O1 : Inport  Port=7  OutDataTypeStr=boolean
  O2 : Inport  Port=8  OutDataTypeStr=boolean
  O4 : Inport  Port=9  OutDataTypeStr=boolean
  LD : Inport  Port=10  OutDataTypeStr=boolean
  CW1C : Inport  Port=11  OutMin=0  OutMax=4  OutDataTypeStr=int8
  CW2C : Inport  Port=12  OutMin=0  OutMax=4  OutDataTypeStr=int8
  CW4C : Inport  Port=13  OutMin=0  OutMax=4  OutDataTypeStr=int8
  Cyber : Subsystem
  M : Memory
  M1 : Memory
  M3 : Memory
  Physical : Subsystem
  S1 : Subsystem
  S2 : Subsystem
  S4 : Subsystem
  W1Pos : Outport
  W2Pos : Outport  Port=2
  W4Pos : Outport  Port=3
  wires:
  Cyber/3(W4) -> Physical/3(InW4)
  DW4/1 -> Cyber/6(DW4)
  Physical/3(W4) -> S4/1(PhyMeasure), W4Pos/1
  DW2/1 -> Cyber/5(DW2)
  P3W4/1 -> Cyber/8(P3W4)
  S2/1(SensorOut) -> M1/1
  Physical/2(W2) -> S2/1(PhyMeasure), W2Pos/1
  DW1/1 -> Cyber/4(DW1)
  M/1 -> Cyber/1(PosW1)
  M1/1 -> Cyber/2(PosW2)
  S4/1(SensorOut) -> M3/1
  CW1C/1 -> Cyber/14(CW1C)
  P1W4/1 -> Cyber/9(P1W4)
  P1W2/1 -> Cyber/7(P1W2)
  Cyber/2(W2) -> Physical/2(InW2)
  Cyber/1(W1) -> Physical/1(InW1)
  O1/1 -> Cyber/10(OW1)
  LD/1 -> Cyber/13(LD)
  O2/1 -> Cyber/11(OW2)
  O4/1 -> Cyber/12(OW4)
  Physical/1(W1) -> S1/1(PhyMeasure), W1Pos/1
  CW4C/1 -> Cyber/16(CW4C)
  CW2C/1 -> Cyber/15(CW2C)
  S1/1(SensorOut) -> M/1
  M3/1 -> Cyber/3(PosW4)

== system c00014M_harness/M116 ==
  DW1 : Inport  OutMin=0  OutMax=4  OutDataTypeStr=int8
  DW2 : Inport  Port=2  OutMin=0  OutMax=4  OutDataTypeStr=int8
  DW4 : Inport  Port=3  OutMin=0  OutMax=4  OutDataTypeStr=int8
  P1W2 : Inport  Port=4  OutMin=0  OutMax=4  OutDataTypeStr=int8
  P3W4 : Inport  Port=5  OutMin=0  OutMax=4  OutDataTypeStr=int8
  P1W4 : Inport  Port=6  OutMin=0  OutMax=4  OutDataTypeStr=int8
  O1 : Inport  Port=7  OutDataTypeStr=boolean
  O2 : Inport  Port=8  OutDataTypeStr=boolean
  O4 : Inport  Port=9  OutDataTypeStr=boolean
  LD : Inport  Port=10  OutDataTypeStr=boolean
  CW1C : Inport  Port=11  OutMin=0  OutMax=4  OutDataTypeStr=int8
  CW2C : Inport  Port=12  OutMin=0  OutMax=4  OutDataTypeStr=int8
  CW4C : Inport  Port=13  OutMin=0  OutMax=4  OutDataTypeStr=int8
  Cyber : Subsystem
  M : Memory
  M1 : Memory
  M3 : Memory
  Physical : Subsystem
  S1 : Subsystem
  S2 : Subsystem
  S4 : Subsystem
  W1Pos : Outport
  W2Pos : Outport  Port=2
  W4Pos : Outport  Port=3
  wires:
  Cyber/3(W4) -> Physical/3(InW4)
  DW4/1 -> Cyber/6(DW4)
  Physical/3(W4) -> S4/1(PhyMeasure), W4Pos/1
  DW2/1 -> Cyber/5(DW2)
  P3W4/1 -> Cyber/8(P3W4)
  S2/1(SensorOut) -> M1/1
  Physical/2(W2) -> S2/1(PhyMeasure), W2Pos/1
  DW1/1 -> Cyber/4(DW1)
  M/1 -> Cyber/1(PosW1)
  M1/1 -> Cyber/2(PosW2)
  S4/1(SensorOut) -> M3/1
  CW1C/1 -> Cyber/14(CW1C)
  P1W4/1 -> Cyber/9(P1W4)
  P1W2/1 -> Cyber/7(P1W2)
  Cyber/2(W2) -> Physical/2(InW2)
  Cyber/1(W1) -> Physical/1(InW1)
  O1/1 -> Cyber/10(OW1)
  LD/1 -> Cyber/13(LD)
  O2/1 -> Cyber/11(OW2)
  O4/1 -> Cyber/12(OW4)
  Physical/1(W1) -> S1/1(PhyMeasure), W1Pos/1
  CW4C/1 -> Cyber/16(CW4C)
  CW2C/1 -> Cyber/15(CW2C)
  S1/1(SensorOut) -> M/1
  M3/1 -> Cyber/3(PosW4)

== system c00014M_harness/M118 ==
  DW1 : Inport  OutMin=0  OutMax=4  OutDataTypeStr=int8
  DW2 : Inport  Port=2  OutMin=0  OutMax=4  OutDataTypeStr=int8
  DW4 : Inport  Port=3  OutMin=0  OutMax=4  OutDataTypeStr=int8
  P1W2 : Inport  Port=4  OutMin=0  OutMax=4  OutDataTypeStr=int8
  P3W4 : Inport  Port=5  OutMin=0  OutMax=4  OutDataTypeStr=int8
  P1W4 : Inport  Port=6  OutMin=0  OutMax=4  OutDataTypeStr=int8
  O1 : Inport  Port=7  OutDataTypeStr=boolean
  O2 : Inport  Port=8  OutDataTypeStr=boolean
  O4 : Inport  Port=9  OutDataTypeStr=boolean
  LD : Inport  Port=10  OutDataTypeStr=boolean
  CW1C : Inport  Port=11  OutMin=0  OutMax=4  OutDataTypeStr=int8
  CW2C : Inport  Port=12  OutMin=0  OutMax=4  OutDataTypeStr=int8
  CW4C : Inport  Port=13  OutMin=0  OutMax=4  OutDataTypeStr=int8
  Cyber : Subsystem
  M : Memory
  M1 : Memory
  M3 : Memory
  Physical : Subsystem
  S1 : Subsystem
  S2 : Subsystem
  S4 : Subsystem
  W1Pos : Outport
  W2Pos : Outport  Port=2
  W4Pos : Outport  Port=3
  wires:
  Cyber/3(W4) -> Physical/3(InW4)
  DW4/1 -> Cyber/6(DW4)
  Physical/3(W4) -> S4/1(PhyMeasure), W4Pos/1
  DW2/1 -> Cyber/5(DW2)
  P3W4/1 -> Cyber/8(P3W4)
  S2/1(SensorOut) -> M1/1
  Physical/2(W2) -> S2/1(PhyMeasure), W2Pos/1
  DW1/1 -> Cyber/4(DW1)
  M/1 -> Cyber/1(PosW1)
  M1/1 -> Cyber/2(PosW2)
  S4/1(SensorOut) -> M3/1
  CW1C/1 -> Cyber/14(CW1C)
  P1W4/1 -> Cyber/9(P1W4)
  P1W2/1 -> Cyber/7(P1W2)
  Cyber/2(W2) -> Physical/2(InW2)
  Cyber/1(W1) -> Physical/1(InW1)
  O1/1 -> Cyber/10(OW1)
  LD/1 -> Cyber/13(LD)
  O2/1 -> Cyber/11(OW2)
  O4/1 -> Cyber/12(OW4)
  Physical/1(W1) -> S1/1(PhyMeasure), W1Pos/1
  CW4C/1 -> Cyber/16(CW4C)
  CW2C/1 -> Cyber/15(CW2C)
  S1/1(SensorOut) -> M/1
  M3/1 -> Cyber/3(PosW4)

== system c00014M_harness/M119 ==
  DW1 : Inport  OutMin=0  OutMax=4  OutDataTypeStr=int8
  DW2 : Inport  Port=2  OutMin=0  OutMax=4  OutDataTypeStr=int8
  DW4 : Inport  Port=3  OutMin=0  OutMax=4  OutDataTypeStr=int8
  P1W2 : Inport  Port=4  OutMin=0  OutMax=4  OutDataTypeStr=int8
  P3W4 : Inport  Port=5  OutMin=0  OutMax=4  OutDataTypeStr=int8
  P1W4 : Inport  Port=6  OutMin=0  OutMax=4  OutDataTypeStr=int8
  O1 : Inport  Port=7  OutDataTypeStr=boolean
  O2 : Inport  Port=8  OutDataTypeStr=boolean
  O4 : Inport  Port=9  OutDataTypeStr=boolean
  LD : Inport  Port=10  OutDataTypeStr=boolean
  CW1C : Inport  Port=11  OutMin=0  OutMax=4  OutDataTypeStr=int8
  CW2C : Inport  Port=12  OutMin=0  OutMax=4  OutDataTypeStr=int8
  CW4C : Inport  Port=13  OutMin=0  OutMax=4  OutDataTypeStr=int8
  Cyber : Subsystem
  M : Memory
  M1 : Memory
  M3 : Memory
  Physical : Subsystem
  S1 : Subsystem
  S2 : Subsystem
  S4 : Subsystem
  W1Pos : Outport
  W2Pos : Outport  Port=2
  W4Pos : Outport  Port=3
  wires:
  Cyber/3(W4) -> Physical/3(InW4)
  DW4/1 -> Cyber/6(DW4)
  Physical/3(W4) -> S4/1(PhyMeasure), W4Pos/1
  DW2/1 -> Cyber/5(DW2)
  P3W4/1 -> Cyber/8(P3W4)
  S2/1(SensorOut) -> M1/1
  Physical/2(W2) -> S2/1(PhyMeasure), W2Pos/1
  DW1/1 -> Cyber/4(DW1)
  M/1 -> Cyber/1(PosW1)
  M1/1 -> Cyber/2(PosW2)
  S4/1(SensorOut) -> M3/1
  CW1C/1 -> Cyber/14(CW1C)
  P1W4/1 -> Cyber/9(P1W4)
  P1W2/1 -> Cyber/7(P1W2)
  Cyber/2(W2) -> Physical/2(InW2)
  Cyber/1(W1) -> Physical/1(InW1)
  O1/1 -> Cyber/10(OW1)
  LD/1 -> Cyber/13(LD)
  O2/1 -> Cyber/11(OW2)
  O4/1 -> Cyber/12(OW4)
  Physical/1(W1) -> S1/1(PhyMeasure), W1Pos/1
  CW4C/1 -> Cyber/16(CW4C)
  CW2C/1 -> Cyber/15(CW2C)
  S1/1(SensorOut) -> M/1
  M3/1 -> Cyber/3(PosW4)

== system c00014M_harness/M120 ==
  DW1 : Inport  OutMin=0  OutMax=4  OutDataTypeStr=int8
  DW2 : Inport  Port=2  OutMin=0  OutMax=4  OutDataTypeStr=int8
  DW4 : Inport  Port=3  OutMin=0  OutMax=4  OutDataTypeStr=int8
  P1W2 : Inport  Port=4  OutMin=0  OutMax=4  OutDataTypeStr=int8
  P3W4 : Inport  Port=5  OutMin=0  OutMax=4  OutDataTypeStr=int8
  P1W4 : Inport  Port=6  OutMin=0  OutMax=4  OutDataTypeStr=int8
  O1 : Inport  Port=7  OutDataTypeStr=boolean
  O2 : Inport  Port=8  OutDataTypeStr=boolean
  O4 : Inport  Port=9  OutDataTypeStr=boolean
  LD : Inport  Port=10  OutDataTypeStr=boolean
  CW1C : Inport  Port=11  OutMin=0  OutMax=4  OutDataTypeStr=int8
  CW2C : Inport  Port=12  OutMin=0  OutMax=4  OutDataTypeStr=int8
  CW4C : Inport  Port=13  OutMin=0  OutMax=4  OutDataTypeStr=int8
  Cyber : Subsystem
  M : Memory
  M1 : Memory
  M3 : Memory
  Physical : Subsystem
  S1 : Subsystem
  S2 : Subsystem
  S4 : Subsystem
  W1Pos : Outport
  W2Pos : Outport  Port=2
  W4Pos : Outport  Port=3
  wires:
  Cyber/3(W4) -> Physical/3(InW4)
  DW4/1 -> Cyber/6(DW4)
  Physical/3(W4) -> S4/1(PhyMeasure), W4Pos/1
  DW2/1 -> Cyber/5(DW2)
  P3W4/1 -> Cyber/8(P3W4)
  S2/1(SensorOut) -> M1/1
  Physical/2(W2) -> S2/1(PhyMeasure), W2Pos/1
  DW1/1 -> Cyber/4(DW1)
  M/1 -> Cyber/1(PosW1)
  M1/1 -> Cyber/2(PosW2)
  S4/1(SensorOut) -> M3/1
  CW1C/1 -> Cyber/14(CW1C)
  P1W4/1 -> Cyber/9(P1W4)
  P1W2/1 -> Cyber/7(P1W2)
  Cyber/2(W2) -> Physical/2(InW2)
  Cyber/1(W1) -> Physical/1(InW1)
  O1/1 -> Cyber/10(OW1)
  LD/1 -> Cyber/13(LD)
  O2/1 -> Cyber/11(OW2)
  O4/1 -> Cyber/12(OW4)
  Physical/1(W1) -> S1/1(PhyMeasure), W1Pos/1
  CW4C/1 -> Cyber/16(CW4C)
  CW2C/1 -> Cyber/15(CW2C)
  S1/1(SensorOut) -> M/1
  M3/1 -> Cyber/3(PosW4)

== system c00014M_harness/M122 ==
  DW1 : Inport  OutMin=0  OutMax=4  OutDataTypeStr=int8
  DW2 : Inport  Port=2  OutMin=0  OutMax=4  OutDataTypeStr=int8
  DW4 : Inport  Port=3  OutMin=0  OutMax=4  OutDataTypeStr=int8
  P1W2 : Inport  Port=4  OutMin=0  OutMax=4  OutDataTypeStr=int8
  P3W4 : Inport  Port=5  OutMin=0  OutMax=4  OutDataTypeStr=int8
  P1W4 : Inport  Port=6  OutMin=0  OutMax=4  OutDataTypeStr=int8
  O1 : Inport  Port=7  OutDataTypeStr=boolean
  O2 : Inport  Port=8  OutDataTypeStr=boolean
  O4 : Inport  Port=9  OutDataTypeStr=boolean
  LD : Inport  Port=10  OutDataTypeStr=boolean
  CW1C : Inport  Port=11  OutMin=0  OutMax=4  OutDataTypeStr=int8
  CW2C : Inport  Port=12  OutMin=0  OutMax=4  OutDataTypeStr=int8
  CW4C : Inport  Port=13  OutMin=0  OutMax=4  OutDataTypeStr=int8
  Cyber : Subsystem
  M : Memory
  M1 : Memory
  M3 : Memory
  Physical : Subsystem
  S1 : Subsystem
  S2 : Subsystem
  S4 : Subsystem
  W1Pos : Outport
  W2Pos : Outport  Port=2
  W4Pos : Outport  Port=3
  wires:
  Cyber/3(W4) -> Physical/3(InW4)
  DW4/1 -> Cyber/6(DW4)
  Physical/3(W4) -> S4/1(PhyMeasure), W4Pos/1
  DW2/1 -> Cyber/5(DW2)
  P3W4/1 -> Cyber/8(P3W4)
  S2/1(SensorOut) -> M1/1
  Physical/2(W2) -> S2/1(PhyMeasure), W2Pos/1
  DW1/1 -> Cyber/4(DW1)
  M/1 -> Cyber/1(PosW1)
  M1/1 -> Cyber/2(PosW2)
  S4/1(SensorOut) -> M3/1
  CW1C/1 -> Cyber/14(CW1C)
  P1W4/1 -> Cyber/9(P1W4)
  P1W2/1 -> Cyber/7(P1W2)
  Cyber/2(W2) -> Physical/2(InW2)
  Cyber/1(W1) -> Physical/1(InW1)
  O1/1 -> Cyber/10(OW1)
  LD/1 -> Cyber/13(LD)
  O2/1 -> Cyber/11(OW2)
  O4/1 -> Cyber/12(OW4)
  Physical/1(W1) -> S1/1(PhyMeasure), W1Pos/1
  CW4C/1 -> Cyber/16(CW4C)
  CW2C/1 -> Cyber/15(CW2C)
  S1/1(SensorOut) -> M/1
  M3/1 -> Cyber/3(PosW4)

== system c00014M_harness/M123 ==
  DW1 : Inport  OutMin=0  OutMax=4  OutDataTypeStr=int8
  DW2 : Inport  Port=2  OutMin=0  OutMax=4  OutDataTypeStr=int8
  DW4 : Inport  Port=3  OutMin=0  OutMax=4  OutDataTypeStr=int8
  P1W2 : Inport  Port=4  OutMin=0  OutMax=4  OutDataTypeStr=int8
  P3W4 : Inport  Port=5  OutMin=0  OutMax=4  OutDataTypeStr=int8
  P1W4 : Inport  Port=6  OutMin=0  OutMax=4  OutDataTypeStr=int8
  O1 : Inport  Port=7  OutDataTypeStr=boolean
  O2 : Inport  Port=8  OutDataTypeStr=boolean
  O4 : Inport  Port=9  OutDataTypeStr=boolean
  LD : Inport  Port=10  OutDataTypeStr=boolean
  CW1C : Inport  Port=11  OutMin=0  OutMax=4  OutDataTypeStr=int8
  CW2C : Inport  Port=12  OutMin=0  OutMax=4  OutDataTypeStr=int8
  CW4C : Inport  Port=13  OutMin=0  OutMax=4  OutDataTypeStr=int8
  Cyber : Subsystem
  M : Memory
  M1 : Memory
  M3 : Memory
  Physical : Subsystem
  S1 : Subsystem
  S2 : Subsystem
  S4 : Subsystem
  W1Pos : Outport
  W2Pos : Outport  Port=2
  W4Pos : Outport  Port=3
  wires:
  Cyber/3(W4) -> Physical/3(InW4)
  DW4/1 -> Cyber/6(DW4)
  Physical/3(W4) -> S4/1(PhyMeasure), W4Pos/1
  DW2/1 -> Cyber/5(DW2)
  P3W4/1 -> Cyber/8(P3W4)
  S2/1(SensorOut) -> M1/1
  Physical/2(W2) -> S2/1(PhyMeasure), W2Pos/1
  DW1/1 -> Cyber/4(DW1)
  M/1 -> Cyber/1(PosW1)
  M1/1 -> Cyber/2(PosW2)
  S4/1(SensorOut) -> M3/1
  CW1C/1 -> Cyber/14(CW1C)
  P1W4/1 -> Cyber/9(P1W4)
  P1W2/1 -> Cyber/7(P1W2)
  Cyber/2(W2) -> Physical/2(InW2)
  Cyber/1(W1) -> Physical/1(InW1)
  O1/1 -> Cyber/10(OW1)
  LD/1 -> Cyber/13(LD)
  O2/1 -> Cyber/11(OW2)
  O4/1 -> Cyber/12(OW4)
  Physical/1(W1) -> S1/1(PhyMeasure), W1Pos/1
  CW4C/1 -> Cyber/16(CW4C)
  CW2C/1 -> Cyber/15(CW2C)
  S1/1(SensorOut) -> M/1
  M3/1 -> Cyber/3(PosW4)

== system c00014M_harness/M124 ==
  DW1 : Inport  OutMin=0  OutMax=4  OutDataTypeStr=int8
  DW2 : Inport  Port=2  OutMin=0  OutMax=4  OutDataTypeStr=int8
  DW4 : Inport  Port=3  OutMin=0  OutMax=4  OutDataTypeStr=int8
  P1W2 : Inport  Port=4  OutMin=0  OutMax=4  OutDataTypeStr=int8
  P3W4 : Inport  Port=5  OutMin=0  OutMax=4  OutDataTypeStr=int8
  P1W4 : Inport  Port=6  OutMin=0  OutMax=4  OutDataTypeStr=int8
  O1 : Inport  Port=7  OutDataTypeStr=boolean
  O2 : Inport  Port=8  OutDataTypeStr=boolean
  O4 : Inport  Port=9  OutDataTypeStr=boolean
  LD : Inport  Port=10  OutDataTypeStr=boolean
  CW1C : Inport  Port=11  OutMin=0  OutMax=4  OutDataTypeStr=int8
  CW2C : Inport  Port=12  OutMin=0  OutMax=4  OutDataTypeStr=int8
  CW4C : Inport  Port=13  OutMin=0  OutMax=4  OutDataTypeStr=int8
  Cyber : Subsystem
  M : Memory
  M1 : Memory
  M3 : Memory
  Physical : Subsystem
  S1 : Subsystem
  S2 : Subsystem
  S4 : Subsystem
  W1Pos : Outport
  W2Pos : Outport  Port=2
  W4Pos : Outport  Port=3
  wires:
  Cyber/3(W4) -> Physical/3(InW4)
  DW4/1 -> Cyber/6(DW4)
  Physical/3(W4) -> S4/1(PhyMeasure), W4Pos/1
  DW2/1 -> Cyber/5(DW2)
  P3W4/1 -> Cyber/8(P3W4)
  S2/1(SensorOut) -> M1/1
  Physical/2(W2) -> S2/1(PhyMeasure), W2Pos/1
  DW1/1 -> Cyber/4(DW1)
  M/1 -> Cyber/1(PosW1)
  M1/1 -> Cyber/2(PosW2)
  S4/1(SensorOut) -> M3/1
  CW1C/1 -> Cyber/14(CW1C)
  P1W4/1 -> Cyber/9(P1W4)
  P1W2/1 -> Cyber/7(P1W2)
  Cyber/2(W2) -> Physical/2(InW2)
  Cyber/1(W1) -> Physical/1(InW1)
  O1/1 -> Cyber/10(OW1)
  LD/1 -> Cyber/13(LD)
  O2/1 -> Cyber/11(OW2)
  O4/1 -> Cyber/12(OW4)
  Physical/1(W1) -> S1/1(PhyMeasure), W1Pos/1
  CW4C/1 -> Cyber/16(CW4C)
  CW2C/1 -> Cyber/15(CW2C)
  S1/1(SensorOut) -> M/1
  M3/1 -> Cyber/3(PosW4)

== system c00014M_harness/M126 ==
  DW1 : Inport  OutMin=0  OutMax=4  OutDataTypeStr=int8
  DW2 : Inport  Port=2  OutMin=0  OutMax=4  OutDataTypeStr=int8
  DW4 : Inport  Port=3  OutMin=0  OutMax=4  OutDataTypeStr=int8
  P1W2 : Inport  Port=4  OutMin=0  OutMax=4  OutDataTypeStr=int8
  P3W4 : Inport  Port=5  OutMin=0  OutMax=4  OutDataTypeStr=int8
  P1W4 : Inport  Port=6  OutMin=0  OutMax=4  OutDataTypeStr=int8
  O1 : Inport  Port=7  OutDataTypeStr=boolean
  O2 : Inport  Port=8  OutDataTypeStr=boolean
  O4 : Inport  Port=9  OutDataTypeStr=boolean
  LD : Inport  Port=10  OutDataTypeStr=boolean
  CW1C : Inport  Port=11  OutMin=0  OutMax=4  OutDataTypeStr=int8
  CW2C : Inport  Port=12  OutMin=0  OutMax=4  OutDataTypeStr=int8
  CW4C : Inport  Port=13  OutMin=0  OutMax=4  OutDataTypeStr=int8
  Cyber : Subsystem
  M : Memory
  M1 : Memory
  M3 : Memory
  Physical : Subsystem
  S1 : Subsystem
  S2 : Subsystem
  S4 : Subsystem
  W1Pos : Outport
  W2Pos : Outport  Port=2
  W4Pos : Outport  Port=3
  wires:
  Cyber/3(W4) -> Physical/3(InW4)
  DW4/1 -> Cyber/6(DW4)
  Physical/3(W4) -> S4/1(PhyMeasure), W4Pos/1
  DW2/1 -> Cyber/5(DW2)
  P3W4/1 -> Cyber/8(P3W4)
  S2/1(SensorOut) -> M1/1
  Physical/2(W2) -> S2/1(PhyMeasure), W2Pos/1
  DW1/1 -> Cyber/4(DW1)
  M/1 -> Cyber/1(PosW1)
  M1/1 -> Cyber/2(PosW2)
  S4/1(SensorOut) -> M3/1
  CW1C/1 -> Cyber/14(CW1C)
  P1W4/1 -> Cyber/9(P1W4)
  P1W2/1 -> Cyber/7(P1W2)
  Cyber/2(W2) -> Physical/2(InW2)
  Cyber/1(W1) -> Physical/1(InW1)
  O1/1 -> Cyber/10(OW1)
  LD/1 -> Cyber/13(LD)
  O2/1 -> Cyber/11(OW2)
  O4/1 -> Cyber/12(OW4)
  Physical/1(W1) -> S1/1(PhyMeasure), W1Pos/1
  CW4C/1 -> Cyber/16(CW4C)
  CW2C/1 -> Cyber/15(CW2C)
  S1/1(SensorOut) -> M/1
  M3/1 -> Cyber/3(PosW4)
